simulink model "Modele_Non_Lineaire"  (R2024a)
settings: Solver=VariableStepAuto  StartTime=0.0  StopTime=3  RelTol=1e-3
undefined symbols (not defined in the file): den_mot_simu, g, L, num_mot_simu, r_arm
settings Model: Creator=Mathys  LastModifiedBy=francoisdesautels
settings RTWCC: GPUComputeCapability=3.5

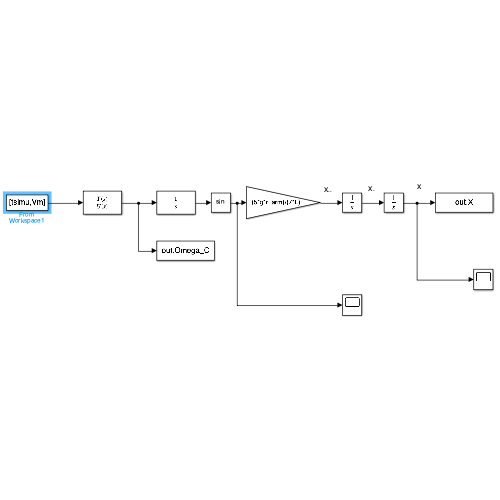
[thumbnail: Simulink's stored preview of the top-level diagram]
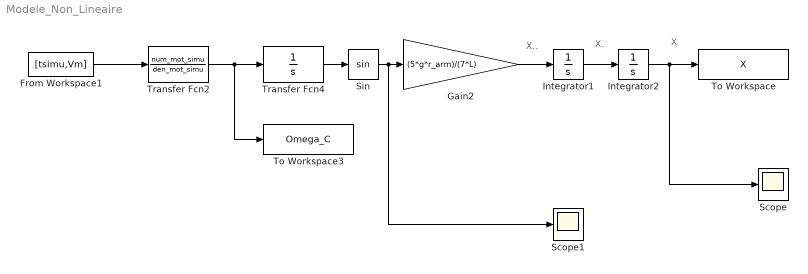
== system Modele_Non_Lineaire ==
  note: X
  note: X.
  note: X..
  From Workspace1 : FromWorkspace  VariableName=[tsimu,Vm]  SampleTime=-1
  Gain2 : Gain  Gain=(5*g*r_arm)/(7*L)
  Integrator1 : Integrator
  Integrator2 : Integrator
  Scope : Scope
  Scope1 : Scope
  Sin : Trigonometry
  To Workspace : ToWorkspace  VariableName=X  SaveFormat=Timeseries  SampleTime=-1
  To Workspace3 : ToWorkspace  VariableName=Omega_C  SampleTime=-1
  Transfer Fcn2 : TransferFcn  Numerator=num_mot_simu  Denominator=den_mot_simu
  Transfer Fcn4 : TransferFcn  Denominator=[1 0]
  wires:
  Sin/1 -> Scope1/1, Gain2/1
  Gain2/1 -> Integrator1/1
  Integrator1/1 -> Integrator2/1
  Integrator2/1 -> Scope/1, To Workspace/1
  Transfer Fcn2/1 -> To Workspace3/1, Transfer Fcn4/1
  From Workspace1/1 -> Transfer Fcn2/1
  Transfer Fcn4/1 -> Sin/1
